simulink model "Motors_Catalogue"  (R2020b)
settings: Solver=VariableStepAuto  StartTime=0.0  StopTime=10.0  RelTol=1e-3
undefined symbols (not defined in the file): Ia_init
settings Model: Creator=mdxavier  LastModifiedBy=mdxavier

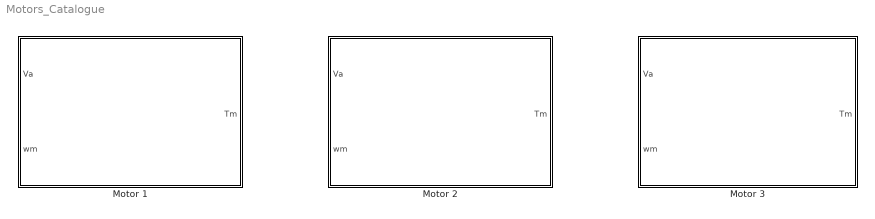
== system Motors_Catalogue ==
  Motor 1 : Subsystem
      mask Display: image('$imagefile'); % Use "Edit Image" on toolstrip to change.
  Motor 2 : Subsystem
      mask Display: image('$imagefile'); % Use "Edit Image" on toolstrip to change.
  Motor 3 : Subsystem
      mask Display: image('$imagefile'); % Use "Edit Image" on toolstrip to change.

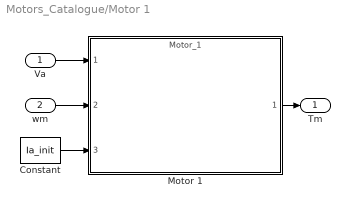
== system Motors_Catalogue/Motor 1 ==
  Va : Inport
  wm : Inport  Port=2
  Constant : Constant  Value=Ia_init
  Motor 1 : ModelReference  ModelNameDialog=Motor_1  ModelReferenceVersion=1.18  CopyOfModelProtected=on
  Tm : Outport
  wires:
  Constant/1 -> Motor 1/3
  Motor 1/1 -> Tm/1
  wm/1 -> Motor 1/2
  Va/1 -> Motor 1/1

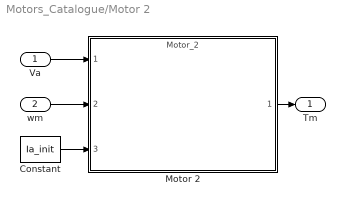
== system Motors_Catalogue/Motor 2 ==
  Va : Inport
  wm : Inport  Port=2
  Constant : Constant  Value=Ia_init
  Motor 2 : ModelReference  ModelNameDialog=Motor_2  ModelReferenceVersion=1.19  CopyOfModelProtected=on
  Tm : Outport
  wires:
  Constant/1 -> Motor 2/3
  wm/1 -> Motor 2/2
  Va/1 -> Motor 2/1
  Motor 2/1 -> Tm/1

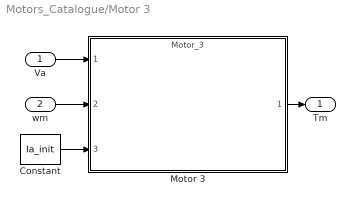
== system Motors_Catalogue/Motor 3 ==
  Va : Inport
  wm : Inport  Port=2
  Constant : Constant  Value=Ia_init
  Motor 3 : ModelReference  ModelNameDialog=Motor_3  ModelReferenceVersion=1.20  CopyOfModelProtected=on
  Tm : Outport
  wires:
  Va/1 -> Motor 3/1
  Constant/1 -> Motor 3/3
  wm/1 -> Motor 3/2
  Motor 3/1 -> Tm/1
